simulink model "DVsimulink"  (R2015a)
settings: Solver=ode45  StartTime=0.0  StopTime=3  RelTol=1e-3
values from neighbouring files (symbols this model uses):
  A = [-14.6713035715  4.37250120377; 876.704382024  -262.351072226]    [Correcteur.mat]    (also in DVinitialisation.m = [[(mufre*cxe-ba-brr)/m nfre*cxe/m];     [-r0*mufre*cxe/Jr -r; Fct_transfer_lineaire.m = [[a1 a2];     a3 a4]; QFT.m = [[(mufre*cxe-ba-brr)/m nu*cxe/m];[-r0*mufre*cxe/J -r0*nu*cxe)
  alpha = 0    [Correcteur.mat]    (also in DVinitialisation.m; PIDF_Design.m = tan((PhiM/Nd+pi/2)/2); QFT.m)
  B = [0 -125]    [Correcteur.mat]    (also in DVinitialisation.m = [0;-K/Jr]; Fct_transfer_lineaire.m = [0;K]; QFT.m = [0;-K/J]; pacejka_BE_Matlab_fnc.m = BCD/(C*D))
  br = 0.001    [Correcteur.mat]    (also in DVinitialisation.m; QFT.m)
  C = [0 1]    [Correcteur.mat]    (also in DVinitialisation.m; Fct_transfer_lineaire.m; QFT.m; pacejka_BE_Matlab_fnc.m = C_0)
  Cm0 = 42.8155296593    [Correcteur.mat]    (also in DVinitialisation.m = r0*FXE+br*W0; QFT.m = r0*FXE+br*W0)
  Cx = 0.5    [Correcteur.mat]    (also in DVinitialisation.m; QFT.m)
  D = 0    [Correcteur.mat]    (also in DVinitialisation.m = [0]; Fct_transfer_lineaire.m = [0]; QFT.m = [0]; QFTsynth.m = max(step(K*Gn/(1+K*G))))
  fx = 0    [Correcteur.mat]    (also in DVinitialisation.m; QFT.m)
  Fz = 1962    [Correcteur.mat]    (also in DVinitialisation.m; QFT.m = m*g; pacejka_BE_Matlab_fnc.m = in(3))
  g = 9.81    [Correcteur.mat]    (also in DVinitialisation.m; QFT.m)
  J = 1    [Correcteur.mat]    (also in DVinitialisation.m; QFT.m)
  K = 125    [Correcteur.mat]    (also in DVinitialisation.m; PIDF_Design.m = K/M; QFT.m)
  lambda0 = 0.0136    [Correcteur.mat]    (also in DVinitialisation.m; QFT.m)
  lambda2 = 4e-08    [Correcteur.mat]    (also in DVinitialisation.m; QFT.m)
  m = 200    [Correcteur.mat]    (also in DVinitialisation.m; QFT.m = var1(i1))
  mu = 1    [Correcteur.mat]    (also in DVinitialisation.m; QFT.m = var2(i2); pacejka_BE_Matlab_fnc.m = in(4))
  muvar = 0.1    [DVinitialisation.m]
  pneu = [1.712 -66.87 1169 851.9 4.943 0.01399 -0.1911 1 0.972 0 0.186 0.22 ... (35 elements, 1x35)]    [Correcteur.mat]    (also in DVinitialisation.m = [a0,a1,a2,a3,a4,a5,a6,a7,am0,am1,am2,am3,am4,am5,am6,am7,am8; pacejka_BE_Matlab_fnc.m = in(5:end); param_pneu_P1_OK.m = [a0,a1,a2,a3,a4,a5,a6,a7,am0,am1,am2,am3,am4,am5,am6,am7,am8)
  r0 = 0.3    [Correcteur.mat]    (also in DVinitialisation.m; QFT.m)
  ro = 1.225    [Correcteur.mat]    (also in DVinitialisation.m; QFT.m)
  Sx = 1    [Correcteur.mat]    (also in DVinitialisation.m; QFT.m)
  VMAX = 55.5555555556    [Correcteur.mat]    (also in DVinitialisation.m; QFT.m)
  VMIN = 0.138888888889    [Correcteur.mat]    (also in DVinitialisation.m; QFT.m)
  Vx0 = 19.4444444444    [Correcteur.mat]    (also in DVinitialisation.m; QFT.m = var3(i3))
  W0 = 64.9781778438    [Correcteur.mat]    (also in DVinitialisation.m = 1/r0*(Vx0/(1-(Te/100))); QFT.m = 1/r0*(Vx0/(1-(Te/100))))
  WMAX = 185.185185185    [Correcteur.mat]    (also in DVinitialisation.m; QFT.m)
  WMIN = 0    [Correcteur.mat]    (also in DVinitialisation.m; QFT.m)
libraries: cstblocks x2, simulink x2
settings Model: Creator=StephaneBarroso  LastModifiedBy=StephaneBarroso

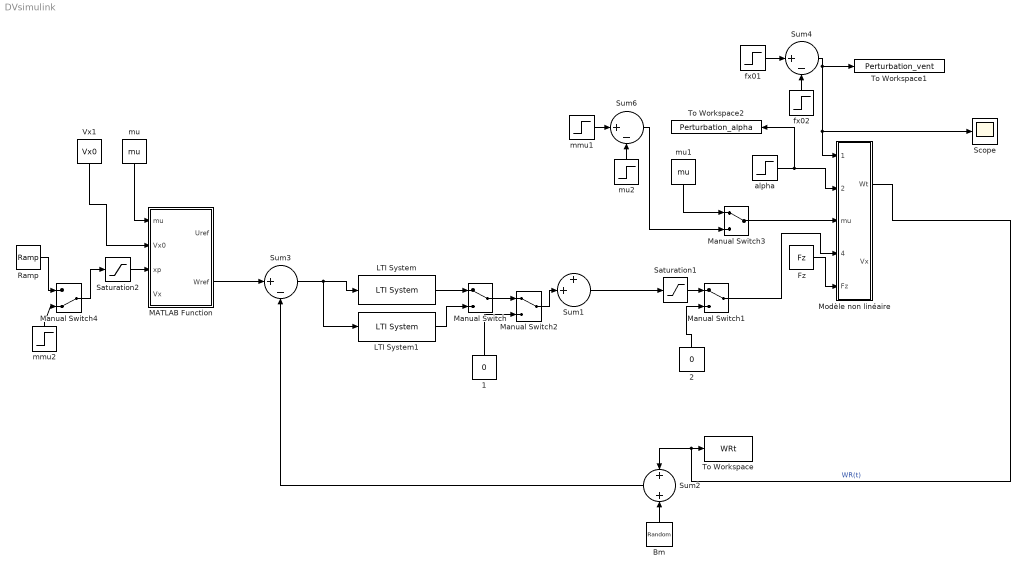
== system DVsimulink ==
  1 : Constant  Value=0
  2 : Constant  Value=0
  Bm : UniformRandomNumber  SampleTime=0
  Fz : Constant  Value=Fz
  LTI System : cstblocks/LTI System  sys=Correcteur  IC=[]
  LTI System1 : cstblocks/LTI System  sys=Co  IC=[]
  MATLAB Function : MATLAB Function  TreatAsAtomicUnit=on
  Manual Switch{,1..3} (4 alike) : ManualSwitch
  Manual Switch4 : ManualSwitch  CurrentSetting=0
  Modèle non linéaire : Subsystem
  Ramp : simulink/Sources/Ramp  slope=2500/Kp/K  start=2.017  X0=0
  Saturation1 : Saturate  UpperLimit=12  LowerLimit=0
  Saturation2 : Saturate  UpperLimit=0.12  LowerLimit=0
  Scope : Scope
      settings: SaveName=ScopeData3
  Sum1 : Sum  Inputs=++|
  Sum2 : Sum
  Sum3 : Sum  Inputs=|+-
  Sum4 : Sum  Inputs=|+-
  Sum6 : Sum  Inputs=|+-
  To Workspace : ToWorkspace  VariableName=WRt  SaveFormat=Timeseries  SampleTime=-1
  To Workspace1 : ToWorkspace  VariableName=Perturbation_vent  SaveFormat=Timeseries  SampleTime=-1
  To Workspace2 : ToWorkspace  VariableName=Perturbation_alpha  SaveFormat=Timeseries  SampleTime=-1
  Vx1 : Constant  Value=Vx0
  alpha : Step  Time=2  After=alpha  SampleTime=0
  fx01 : Step  Time=2.5  After=fx  SampleTime=0
  fx02 : Step  Time=3.5  After=fx  SampleTime=0
  mmu1 : Step  Time=3  Before=mu  After=muvar  SampleTime=0
  mmu2 : Step  Time=0.3  After=0.01  SampleTime=0
  mu : Constant  Value=mu
  mu1 : Constant  Value=mu
  mu2 : Step  Time=4  After=-mu+muvar  SampleTime=0
  wires:
  fx01/1 -> Sum4/1
  fx02/1 -> Sum4/2
  Sum4/1 -> Modèle non linéaire/1(Fox), Scope/1, To Workspace1/1
  alpha/1 -> To Workspace2/1, Modèle non linéaire/2("alpha ")
  Sum2/1 -> Sum3/2
  Modèle non linéaire/1(Wt) -> Sum2/1, To Workspace/1  "WR(t)"
  Fz/1 -> Modèle non linéaire/5("Fz ")
  Bm/1 -> Sum2/2
  MATLAB Function/2(Wref) -> Sum3/1
  LTI System/1 -> Manual Switch/1
  LTI System1/1 -> Manual Switch/2
  Sum1/1 -> Saturation1/1
  Saturation1/1 -> Manual Switch1/1
  Saturation2/1 -> MATLAB Function/3(xp)
  Vx1/1 -> MATLAB Function/2(Vx0)
  mu/1 -> MATLAB Function/1(mu)
  Sum3/1 -> LTI System1/1, LTI System/1
  Manual Switch1/1 -> Modèle non linéaire/4("Uct ")
  1/1 -> Manual Switch2/2
  Manual Switch/1 -> Manual Switch2/1
  Manual Switch2/1 -> Sum1/2
  mmu1/1 -> Sum6/1
  mu2/1 -> Sum6/2
  Manual Switch3/1 -> Modèle non linéaire/3("mu ")
  mu1/1 -> Manual Switch3/1
  Sum6/1 -> Manual Switch3/2
  Ramp/1 -> Manual Switch4/1
  Manual Switch4/1 -> Saturation2/1
  2/1 -> Manual Switch1/2
  mmu2/1 -> Manual Switch4/2

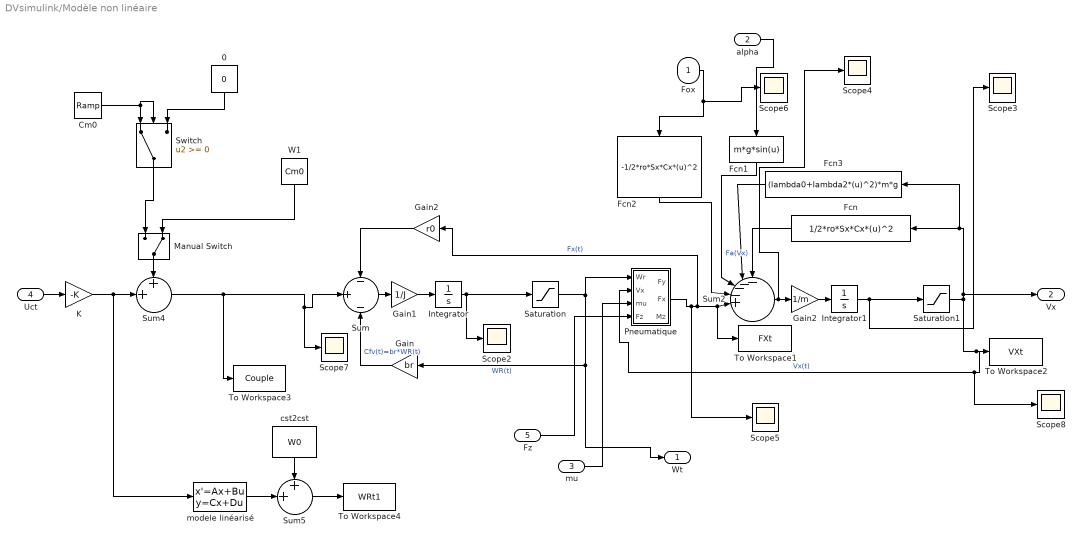
== system DVsimulink/Modèle non linéaire ==
  Fox : Inport
  "alpha " : Inport  Port=2
  "mu " : Inport  Port=3
  "Uct " : Inport  Port=4
  "Fz " : Inport  Port=5
  "0 " : Constant  Value=0
  Cm0 : simulink/Sources/Ramp  slope=-2500  start=2  X0=Cm0
  Fcn : Fcn  Expr=1/2*ro*Sx*Cx*(u)^2
  Fcn1 : Fcn  Expr=m*g*sin(u)
  Fcn2 : Fcn  Expr=-1/2*ro*Sx*Cx*(u)^2
  Fcn3 : Fcn  Expr=(lambda0+lambda2*(u)^2)*m*g
  Gain : Gain  Gain=br
  Gain1 : Gain  Gain=1/J
  Gain2 : Gain  Gain=r0
  "Gain2 " : Gain  Gain=1/m
  Integrator : Integrator  InitialCondition=W0
  Integrator1 : Integrator  InitialCondition=Vx0
  K : Gain  Gain=-K
  Manual Switch : ManualSwitch  CurrentSetting=0
  Pneumatique : Subsystem
  Saturation : Saturate  UpperLimit=WMAX  LowerLimit=WMIN
  Saturation1 : Saturate  UpperLimit=VMAX  LowerLimit=VMIN
  Scope{2..8} (7 alike) : Scope
      Scope2 settings: SaveName=ScopeData2
      Scope3 settings: SaveName=ScopeData6
      Scope4 settings: SaveName=ScopeData4
      Scope5 settings: SaveName=ScopeData7
      Scope6 settings: SaveName=ScopeData10
      Scope7 settings: YMin=-35  YMax=45  SaveName=ScopeData9
      Scope8 settings: SaveName=ScopeData19
  Sum : Sum  Inputs=-|+|-
  Sum2 : Sum  Inputs=----+|||
  Sum4 : Sum  Inputs=++|
  Sum5 : Sum  Inputs=++|
  Switch : Switch
  To Workspace1 : ToWorkspace  VariableName=FXt  SaveFormat=Timeseries  SampleTime=-1
  To Workspace2 : ToWorkspace  VariableName=VXt  SaveFormat=Timeseries  SampleTime=-1
  To Workspace3 : ToWorkspace  VariableName=Couple  SaveFormat=Timeseries  SampleTime=-1
  To Workspace4 : ToWorkspace  VariableName=WRt1  SaveFormat=Timeseries  SampleTime=-1
  W1 : Constant  Value=Cm0
  "cst2cst " : Constant  Value=W0
  modele linéarisé : StateSpace  A=A  B=B  C=C  D=D  X0=0
  Wt : Outport
  "Vx " : Outport  Port=2
  wires:
  Pneumatique/2(Fx) -> Scope5/1, Gain2/1, To Workspace1/1, Sum2/5  "Fx(t)"
  "Uct "/1 -> K/1
  Sum/1 -> Gain1/1
  Fcn/1 -> Sum2/1  "Fa(Vx)"
  Sum2/1 -> Scope4/1, "Gain2 "/1
  Fcn3/1 -> Sum2/2
  Fcn2/1 -> Sum2/4
  Integrator1/1 -> Saturation1/1, Scope3/1
  Gain/1 -> Sum/3  "Cfv(t)=br*WR(t)"
  "Gain2 "/1 -> Integrator1/1
  Fox/1 -> Scope6/1, Fcn2/1
  Fcn1/1 -> Sum2/3
  "alpha "/1 -> Fcn1/1
  Saturation1/1 -> "Vx "/1, Fcn3/1, Fcn/1, To Workspace2/1, Scope8/1, Pneumatique/2(Vx)  "Vx(t)"
  Gain1/1 -> Integrator/1
  Integrator/1 -> Saturation/1, Scope2/1
  Saturation/1 -> Wt/1, Gain/1, Pneumatique/1(Wr)  "WR(t)"
  Gain2/1 -> Sum/1
  "mu "/1 -> Pneumatique/3("mu ")
  "Fz "/1 -> Pneumatique/4("Fz ")
  K/1 -> modele linéarisé/1, Sum4/2
  Cm0/1 -> Switch/2, Switch/1
  "0 "/1 -> Switch/3
  Switch/1 -> Manual Switch/1
  Manual Switch/1 -> Sum4/1
  W1/1 -> Manual Switch/2
  Sum4/1 -> To Workspace3/1, Scope7/1, Sum/2
  Sum5/1 -> To Workspace4/1
  modele linéarisé/1 -> Sum5/2
  "cst2cst "/1 -> Sum5/1

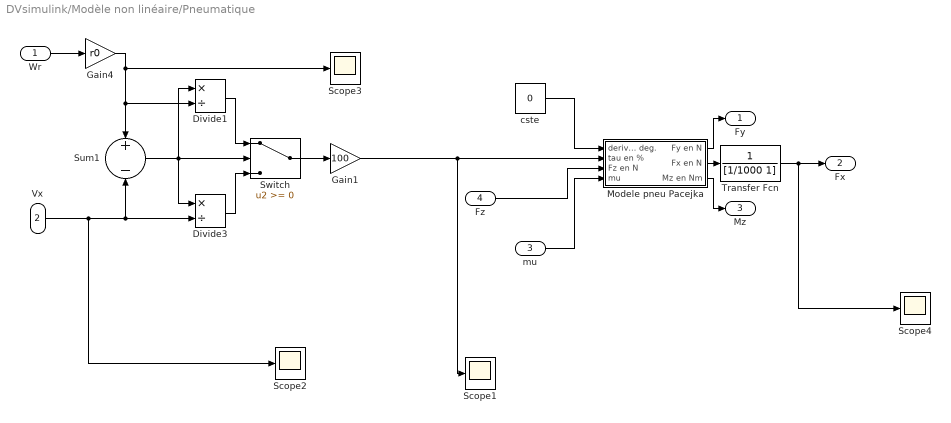
== system DVsimulink/Modèle non linéaire/Pneumatique ==
  Wr : Inport
  Vx : Inport  Port=2
  "mu " : Inport  Port=3
  "Fz " : Inport  Port=4
  Divide1 : Product  Inputs=*/
  Divide3 : Product  Inputs=*/
  Gain1 : Gain  Gain=100
  Gain4 : Gain  Gain=r0
  Modele pneu Pacejka : Subsystem
  Scope{1..4} (4 alike) : Scope
      Scope1 settings: SaveName=ScopeData5
      Scope4 settings: SaveName=ScopeData8
  Sum1 : Sum  Inputs=+-
  Switch : Switch
  Transfer Fcn : TransferFcn  Denominator=[1/1000 1]
  cste : Constant  Value=0
  Fy : Outport
  Fx : Outport  Port=2
  Mz : Outport  Port=3
  wires:
  "Fz "/1 -> Modele pneu Pacejka/3(Fz en N)
  "mu "/1 -> Modele pneu Pacejka/4(mu)
  Gain4/1 -> Scope3/1, Divide1/2, Sum1/1
  Modele pneu Pacejka/3(Mz en Nm) -> Mz/1
  Modele pneu Pacejka/2(Fx en N) -> Transfer Fcn/1
  Modele pneu Pacejka/1(Fy en N) -> Fy/1
  Vx/1 -> Scope2/1, Divide3/2, Sum1/2
  Transfer Fcn/1 -> Scope4/1, Fx/1
  Wr/1 -> Gain4/1
  cste/1 -> Modele pneu Pacejka/1(deriv. en deg.)
  Sum1/1 -> Divide3/1, Divide1/1, Switch/2
  Divide1/1 -> Switch/1
  Divide3/1 -> Switch/3
  Gain1/1 -> Modele pneu Pacejka/2(tau en %), Scope1/1
  Switch/1 -> Gain1/1

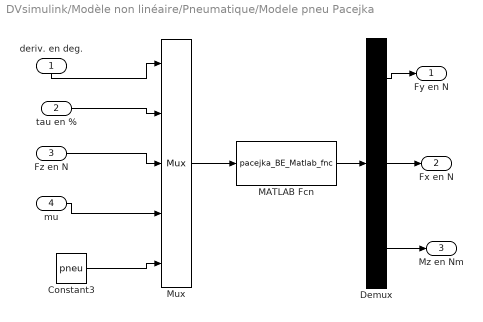
== system DVsimulink/Modèle non linéaire/Pneumatique/Modele pneu Pacejka ==
  deriv. en deg. : Inport
  tau en % : Inport  Port=2
  Fz en N : Inport  Port=3
  mu : Inport  Port=4
  Constant3 : Constant  Value=pneu
  Demux : Demux  Outputs=3
  MATLAB Fcn : MATLABFcn  MATLABFcn=pacejka_BE_Matlab_fnc  OutputDimensions=3
  Mux : Mux  Inputs=5
  Fy en N : Outport
  Fx en N : Outport  Port=2
  Mz en Nm : Outport  Port=3
  wires:
  MATLAB Fcn/1 -> Demux/1
  Mux/1 -> MATLAB Fcn/1
  deriv. en deg./1 -> Mux/1
  Demux/1 -> Fy en N/1
  Demux/2 -> Fx en N/1
  Demux/3 -> Mz en Nm/1
  tau en %/1 -> Mux/2
  Fz en N/1 -> Mux/3
  mu/1 -> Mux/4
  Constant3/1 -> Mux/5

== matlab function DVsimulink/MATLAB Function ==
  data: mu input; Vx0 input; Uref output; xp input; Wref output; Vx input
function [Uref,Wref] = fcn(mu,Vx0,xp,Vx)
%#codegen

J=1;             %Kg.m2      Inertie roue
br=1e-3;        %Nm.s/rad   Coefficient de frottement visqueux
r0=0.3 ;         %m          Rayon de la roue sous charge
Sx=1;            %m2         Surface projetée longitudinalment pour 1/4 du véhicule
Cx=0.5;          %           Coefficient de trainée longitudinale
ro=1.225;        %kg/m3      Masse volumique de l'air
lambda0=13.6e-3;   %s/m2       Constante de la résistance au roulement
lambda2=4e-8; %s/m2       Constante de la résistance au roulement
K=125;           %Nm/V       Gain statique de l actionneur EMB
Kp=100;          %V/m        Gain statique de la pedale de frein
cp=0.12;         %m          Course de la pérale de frein
m=200;           %kg         Masse du 1/4 de véhicule
g=9.81;            %Nm/kg      Gravite
Fz=m*g;         %N

b3 = 23.9;
b4 = 242;
b5 = 0;
Z=Fz*1e-3;

cx=mu*(b3*Z^2+b4*Z)*exp(-b5*Z); % N/%
%cx=Bx*Cx*Dx;
%% état initial

FAE=1/2*ro*Sx*Cx*Vx0^2;
Frr=(lambda0+lambda2*Vx0^2)*m*g;
FXE=FAE+Frr;
Te=1/cx*FXE;


Topt=0.10;
if xp>0
%Wref=1/r0*(Vx*(1-(Topt)));
Wref=xp;
else
   Wref=1/r0*(Vx0/(1-(Te/100)));
end
Uref=Kp*xp;
